simulink model "Vehicle_Model_Controller_Feb20"  (R2020b)
settings: Solver=VariableStepAuto  StartTime=0.0  StopTime=60  FixedStep=0.015  MaxStep=0.015  RelTol=1e-3
model workspace (MAT data in the model file):
  Kp = 10
  understeer_gradient = 0.05
values from neighbouring files (symbols this model uses):
  I = s3    [optimize_controller.m]    (also in parallel_sim.m)
  P = s2    [optimize_controller.m]    (also in parallel_sim.m)
  T = t_vary(k)    [optimize_controller.m]    (also in parallel_sim.m = T_all(k))
undefined symbols (not defined in the file or in its folder): DiscIntNeverNeededParam
libraries: fl_lib x32, nesl_utility x24, sdl_lib x8, vehdynlibsteering x1, autolibshared x1, autolibdatasheetbattery x1
(part 3 of 3)

== matlab function Vehicle_Model_Controller_Feb20/Driver Input Logic/Torque Vectoring Controller/LP_Calc  ==
  settings: updateMethod=DISCRETE
  data: Tx_actual output double; Tx_fmincon output; prev_torque input; driver_input input; power_limit_battery input; FY input; omega_m input; x input; y input; T2F input; slip_limit input; power_limit input; tau_limit_upper input; tau_limit_lower input; rpm_limit input; omega_m output; lb output single; PID input; ub output single; Aeq output single; beq output single; A output single; b output single; M_max output double; J_z data_store_memory; motor_efficiency data_store_memory; motor_limit_torque data_store_memory; min_speed_regen data_store_memory; power output double; yaw_accel output double; power_fmincon output; yaw_accel_fmincon output; exitflag1 output; exitflag2 output; bigM_flag output; A_bigM output; b_bigM output; c_bigM output; inq_bigM output
function [Tx_actual, Tx_fmincon, omega_m, lb, ub, Aeq, beq, A, b, M_max, power, yaw_accel, power_fmincon, yaw_accel_fmincon, exitflag1, exitflag2, bigM_flag, A_bigM,b_bigM,c_bigM,inq_bigM] = LP_calc(prev_torque, driver_input, power_limit_battery, FY, omega_m, x, y, T2F, slip_limit, power_limit, tau_limit_upper, tau_limit_lower, rpm_limit, PID)
%% LP_calc Computation
% Developer(s):    David Farell
%                  Demetrius Gulewicz
%                  Elliot Stockwell
%                  Tao Sun
%
% Developed for: Purdue Electric Racing
% Date:          12/25/2021
%
% Description: This function primarily computes the desired torque
%              distribution after constructing an optimization statement.
%
%
%% Pass Through Signals
% omega_m - Motor Shaft Angular Velocity [rad/s][1x4]
%
%
%% Input Only
% prev_torque - Torque Requested To Motor In Previous Time Step [Nm][4x1]
% driver_input - Proportion of total available power to use [Unitless][1x1]
% T2F - Convert Torque At The Motor Shaft to Force At The Tire [1/m][1x4]
% power_limit_battery - Max & Min Total Battery Power Output [W][1x2]
% FY - Tires Forces y Direction, Tire fixed coordinates [N][1x4]
% x - Equivalent Distances That FX Acts From CoG [m][1x4]
% y - Equivalent Distances That FY Acts From CoG [m][1x4]
% slip_limit - Max Torque Before Tire Slips [Nm][1x4]
% torque_limit_motor - Max Torque Motor Can Output [Nm][1x4]
% tau_limit_upper - Max Torque Motor Is Allowed To Change To [Nm][1x4]
% tau_limit_lower - Min Torque Motor Is Allowed To Change To [Nm][1x4]
% PID - Desired Yaw Acceleration [rad/s^2][1x1]
%
%
%% Output Only
% Tx - Torque Request To Motors [Nm][4x1]
% lb - Min Torque Request [Nm][1x4]
% ub - Max Torque Request [Nm][1x4]
% Aeq - Moment About CoG, Optimization Variable [rad/s^2][1x1]
% beq - Moment About CoG, Yaw Acceleration & Other Foces [rad/s^2][1x1]
% A - Power Consumed, Optimization Variable [W][1x1]
% b - Power Consumed, Driver Input [W][1x1]
% M_max - Max & Min Yaw Acceleration Achievable With lb & ub [rad/s^2][1x2]
% Power - Total Estimated Power Consumed by the 4 Motors
% TR - The Estimated Yaw Acceleration from the Vehicle
%
%
%% Constants
global J_z; % Polar Moment Of Inertia [kg m^2][1x1]
global motor_efficiency; % Motor efficiency [Unitless][1x4]
global motor_limit_torque; % Minimum & Max Torque Request From Motor [Nm][1x2]
global min_speed_regen; % Min Motor Shaft Speed For Regen Braking [rad/s][1x1]


%% Calculation
% Calculate Boundary Conditions, The Max and Min Allowable Torque
ub = single([0, 0, 0, 0]);
lb = single([0, 0, 0, 0]);

for i = 1:4
    ub(i) = min([slip_limit(i), power_limit(i), motor_limit_torque(2), tau_limit_upper(i), rpm_limit(i)]);
    lb(i) = max([-slip_limit(i), -power_limit(i), motor_limit_torque(1), tau_limit_lower(i)]);
end

% Enforce No Backwards Rotation Of Tires
for i = 1:4
   if omega_m(i) < min_speed_regen && lb(i) < -0.1
       lb(i) = -0.001;
   end
end

% Max & Min Forces on the Tires
ub_f = ub .* T2F;
lb_f = lb .* T2F;

% Find Max & Min For PID, The Yaw Acceleration Of The Car
M_max=zeros(1,2);
M_max(1) = (x(1)*ub_f(1)+x(3)*ub_f(3)+x(2)*lb_f(2)+x(4)*lb_f(4)+sum(y.*FY))/J_z;
M_max(2) = (x(2)*ub_f(2)+x(4)*ub_f(4)+x(1)*lb_f(1)+x(3)*lb_f(3)+sum(y.*FY))/J_z;

% Limit PID To Be No Larger Than Possible Due To Torque Constraints
if PID >= M_max(1)
    PID = M_max(1);
elseif PID <= M_max(2)
    PID = M_max(2);
end

% Calculate Yaw Constraint
Aeq = ((1 ./ J_z) .* x) .* T2F;
beq = single(PID-sum(((1 / J_z) * y) .* FY));

% Calculate Power Constraint
if driver_input >=0
    Ac = single([(omega_m ./ motor_efficiency); -(omega_m ./ motor_efficiency)]);
    bc = single([driver_input*power_limit_battery, 0]);
%       A = single(omega_m ./ motor_efficiency);
%       b = single(driver_input*power_limit_battery);
else 
    Ac = single([-(omega_m ./ motor_efficiency); (omega_m ./ motor_efficiency)]);
    bc = single([driver_input*power_limit_battery, 0]);
%       A = single(-omega_m ./ motor_efficiency);
%       b = single(driver_input*power_limit_battery);
end



%% Optimization
% Set Optimization Parameters
options = optimoptions('fmincon','Algorithm','sqp');

Ad = double(Ac);
bd = double(bc);
Aeqd = double(Aeq);
beqd = double(beq);
lbd = double(lb);
ubd = double(ub);

% Determine correct objective function maximize the forces acting on the car
if driver_input >= 0
    objfun = @(q) -sum(q .* double(T2F));
    [Txd1,fval,exitflag1,output] = fmincon(objfun,double(prev_torque'),Ad,bd,Aeqd,beqd,lbd,ubd,[],options);
else 
    objfun = @(q) sum(q .* double(T2F));    
    [Txd1,fval,exitflag1,output] = fmincon(objfun,double(prev_torque'),Ad,bd,Aeqd,beqd,lbd,ubd,[],options);
end 

objfun = @(q) abs(double(PID-(sum(x.*T2F.*q)+sum(y.*FY))/J_z));
[Txd2,fval,exitflag2,output] = fmincon(objfun,double(prev_torque'),Ad,bd,Aeqd,beqd,lbd,ubd,[],options);

Tx_fmincon = Txd1';
if exitflag1 < 0
    Tx_fmincon = Txd2';
end

yaw_accel_fmincon = double((sum(x.*T2F.*Tx_fmincon')+sum(y.*FY))/J_z);

% Compute Requested Power
power_fmincon = double(sum(Tx_fmincon' .* omega_m));


% if exitflag < 0
%     Tx_fmincon = prev_torque;
% %    if (yaw_accel_fmincon > 0)
% %        if yaw_accel_fmincon < PID
% %            Tx_fmincon = double([ub(1) lb(2) ub(3) lb(4)]');
% %            Tx_fmincon = Tx_fmincon - (Tx_fmincon .* 0.2);
% %        elseif yaw_accel_fmincon > PID
% %            Tx_fmincon = double([lb(1) ub(2) lb(3) ub(4)]');
% %            Tx_fmincon = Tx_fmincon + (Tx_fmincon .* 0.2);
% %        end
% %    elseif (yaw_accel_fmincon < 0)
% %        if yaw_accel_fmincon < PID
% %            Tx_fmincon = double([ub(1) lb(2) ub(3) lb(4)]');
% %            Tx_fmincon = Tx_fmincon - (Tx_fmincon .* 0.2);
% %        elseif yaw_accel_fmincon > PID
% %            Tx_fmincon = double([lb(1) ub(2) lb(3) ub(4)]'); 
% %            Tx_fmincon = Tx_fmincon + (Tx_fmincon .* 0.2);
% %        end  
% %    end
% end

%% Optimization
if driver_input >=0
%     A = single([(omega_m ./ motor_efficiency); -(omega_m ./ motor_efficiency)]);
%     b = single([driver_input*power_limit_battery, 0]);
      A = single(omega_m ./ motor_efficiency);
      b = single(driver_input*power_limit_battery);
else 
%     A = single([-(omega_m ./ motor_efficiency); (omega_m ./ motor_efficiency)]);
%     b = single([driver_input*power_limit_battery, 0]);
      A = single(-omega_m ./ motor_efficiency);
      b = single(driver_input*power_limit_battery);
end


% input
% T2F, A, Aeq, lb, ub   [1 * 4] double matrix
% b, A                  double
%
% output
% Tx                    [1 * 4] double matrix, torque output
% flag                  int, -1 = default output
%                             0 = infeasible
%                             1 = max interation reached (20)
%                             2 = problem is unbounded
%                             3 = optimal solution !!!

% setup
Tx_sign = [1, 1, 1, 1]; % 1 = positive, - 1 = negative

c_bigM=[T2F(1), T2F(2), T2F(3), T2F(4)]';
b_bigM=[b, beq, lb(1), lb(2), lb(3), lb(4), ...
    ub(1), ub(2), ub(3), ub(4)]';
A_bigM=[A(1), A(2), A(3), A(4); ...
        Aeq(1), Aeq(2), Aeq(3), Aeq(4); ...
        1, 0, 0, 0; ...
        0, 1, 0, 0; ...
        0, 0, 1, 0; ...
        0, 0, 0, 1; ...
        1, 0, 0, 0; ...
        0, 1, 0, 0; ...
        0, 0, 1, 0; ...
        0, 0, 0, 1];

inq_bigM=[-1, 0, 1, 1, 1, 1, -1, -1, -1, -1];

% detect Tx that are surely negative, negate them
for j = 1:4
    if((b_bigM(j+2) < 0) && (b_bigM(j+6) < 0))
       b_bigM(j+2)      = - b_bigM(j+2);
       b_bigM(j+6)      = - b_bigM(j+6);
       c_bigM(j)        = - c_bigM(j);
       A_bigM(1, j)     = - A_bigM(1, j);
       A_bigM(2, j)     = - A_bigM(2, j);
       inq_bigM(j+2)    = - 1;
       inq_bigM(j+6)    =   1;
       Tx_sign(j)       = - 1;
    end
end

% construct Tableau
p = bigM(A_bigM,b_bigM,c_bigM,inq_bigM,'max');
% solve Tableau
[Tx, bigM_flag] = p.solve; 

% negate back
for j = 1:4
    if(Tx_sign(j) == -1)
        Tx(j) = - Tx(j);
    end
end

                        
                        
%% Extras
% Determine Tracking Signal
Tx_actual = Tx';

if bigM_flag == 0
    Tx_actual = Txd2';
end
Tx_actual = Txd2';
yaw_accel = double((sum(x.*T2F.*Tx_actual')+sum(y.*FY))/J_z);

% Compute Requested Power
power = double(sum(Tx_actual' .* omega_m));

end

== matlab function Vehicle_Model_Controller_Feb20/Motor and Battery/Motors/   ==
  data: Battery_Voltage input; ang_vel_RAD input; battery_current output; Motor_torque input; battery_power output
function [battery_current, battery_power]= get_batt_curr(Battery_Voltage, ang_vel_RAD, Motor_torque)
%% Current Draw
% Developers:    Demetrius Gulewicz

% Developed for: Purdue Electric Racing
% Date:          09/18/2021
%
% Definitions:
% ang_vel_RAD:   Angular velocity of each wheel on the wheel fixed y axis [RAD]
% Motor_torque:  Torque the motor actually outputs                 [Ncm]
% Battery_Voltage: The voltage of the battery                      [V]

%% Definitions
a = 0.0411;
b = 2.7976;
c = 45.978;

t = Motor_torque;
w = ang_vel_RAD;
v = Battery_Voltage;

e = 85;

%% Calculate Current Draw
%x0 = [20, 20, 20, 20];
%options = optimoptions('fsolve','Algorithm','Levenberg-Marquardt');
%F = @(x) ([(a * x(1)^3) + (b * x(1)^2) + (c * x(1)), ] .* v) - (t .* w);
%battery_current = sum(fsolve(F,x0,options));

battery_current = sum((t .* w') ./ (e .* v));
battery_power = battery_current * Battery_Voltage;
end

== matlab function Vehicle_Model_Controller_Feb20/Driver Input Logic/Torque Vectoring Controller/Layer 1 ==
  data: driver_input output; power_limits_battery output; center_steer_angle output; acker_steer_angles output; FY output; omega_w output; T2F output single; T_brake output size=[1 4]; yaw output; yaw_ref output; driver_input input; power_limits_battery input; omega_w input; center_steer_angle input; acker_steer_angles input; FY input size=[1 4]; Vg input; yaw input; K_u data_store_memory; gr data_store_memory; gearbox_efficiency data_store_memory; tau data_store_memory; c_factor data_store_memory; J_z data_store_memory; l data_store_memory; s data_store_memory; r data_store_memory; g data_store_memory; tire_mu data_store_memory; brakeforce_max data_store_memory; brakepad_mu data_store_memory; disk_diameter data_store_memory; mech_brake data_store_memory
function [driver_input, power_limits_battery, center_steer_angle, acker_steer_angles, FY, omega_w, T2F, T_brake, yaw, yaw_ref] = Layer_1(driver_input, power_limits_battery, omega_w, center_steer_angle, acker_steer_angles, FY, Vg, yaw)
%% Layer 1 Computation
% Developer(s):    David Farell
%                  Demetrius Gulewicz
%                  Elliot Stockwell
%                  Tao Sun
%
% Developed for: Purdue Electric Racing
% Date:          12/25/2021
%
% Description: This function primarily computes the reference yaw rate, 
%              and the brake forces & distribution.
%
%
%% Pass Through Signals
% driver_input - Proportion Of Total Available Power To Use [Unitless][1x1]
% power_limits_battery - Max & Min Total Battery Power Output [W][2x1]
% center_steer_angle - Steering Column Angle From Neutral [rad][1x1]
% acker_steer_angles - Angle Tires Are Turned From Neutral [rad][2x1]
% FY - Tires Forces y Direction, Tire Fixed Coordinates [N][1x4]
% omega_w - Angular Velocity Of Tires, Tire Fixed Coordinates [m/s][1x4]
% yaw - Yaw Rate z Direction, Vehicle Fixed Coordinates  [rad/s][1x1]
%
%
%% Input Only
% Vg - Center Of Gravity Velocity, Vehicle Fixed Coordinates [m/s][1x2]
%
%
%% Output Only
% T2F - Convert Torque At The Motor Shaft to Force At The Tire [1/m][1x4]
% T_brake - Mechanical Brake Torque On Each Tire [Nm][1x4]
% yaw_ref - The Desired & Max Allowed Yaw Rate [rad/s][1x2]
%
%
%% Constants
global g; % Acceleration Due To Gravity [m/s^2][1x1]
global tire_mu; % Maximum Friction Coefficient [Unitless][1x4]
global gr; % Gear ratios [Unitless][1x4]
global gearbox_efficiency; % Gearbox Power Transmission Efficiency [Unitless][1x4]
global r; % Tire Radius [m][1x1]
global l; % Wheelbase [m][1x2]
global K_u; % Understeer Gradient [rad/m/s^2][1x1]
global c_factor; % Max Yaw Equation Contributing Factor [Unitless][1x1]
global brakeforce_max; % Max Force Brakes Can Exert On Each Tire Axle [N][1x4]
global brakepad_mu; % Brakepad Friction Coefficient[Unitless][1x1]
global mech_brake; % Value Of driver_input Where Mechanical Braking Begins [Unitless][1x1]
global disk_diameter; % Diameter of brake disk [m][1x1]


%% Calculation
% Convert Torque At The Motor Shaft to Force At The Wheel
% During Runtime, T2F Is Constant
T2F = single((gr .* gearbox_efficiency) ./ r);

% Yaw Calculations
% If yaw_des or yaw_max ever exceed 2, then the exact value is no longer
% needed. As in, the ceiling of these two variables is 2.
v_cog = norm(Vg);
yaw_des = (v_cog * abs(center_steer_angle)) / ((l(1) + l(2)) + (K_u * v_cog ^ 2));
yaw_max = (c_factor * max(tire_mu) * g) / (v_cog);

% Control For Large Max Yaw, For Better Viewing
if yaw_max > 0.7
    yaw_max = 0.7;
end

yaw_ref = [yaw_des, yaw_max];

% Compute brake force and distribution
% for small brakes (input >= mech_brake), only regen braking
% for large brakes (input <= mech_brake), regen & mechanical braking
% note: actual force may not be proportional to the input
T_brake = [0,0,0,0];

if driver_input <= mech_brake   
    brakeforce_ratio = [1, 1, 1, 1] .* -(driver_input - mech_brake) / (1 + mech_brake);
    T_brake = -1.*brakeforce_ratio.*brakeforce_max.*brakepad_mu.*disk_diameter;
    driver_input = -1;
end

if Vg(1) < 0
    T_brake = -T_brake;
end

if abs(Vg(1)) < 0.1
   T_brake = [0 0 0 0]; 
end

if driver_input <= 0 && driver_input >= mech_brake
    driver_input = -driver_input / mech_brake;  % in scale of [-1,0]
end

end
